simulink model "MAPH_Test"  (R2016a)
settings: Solver=FixedStepDiscrete  StartTime=0.0  StopTime=16  FixedStep=0.005  RelTol=1e-3
undefined symbols (not defined in the file): sigbuilder_block
libraries: MAPH x1
settings Model: Creator=oelkawok  LastModifiedBy=oelkawok
settings DataIOCC: SaveOutput=off  SaveTime=off

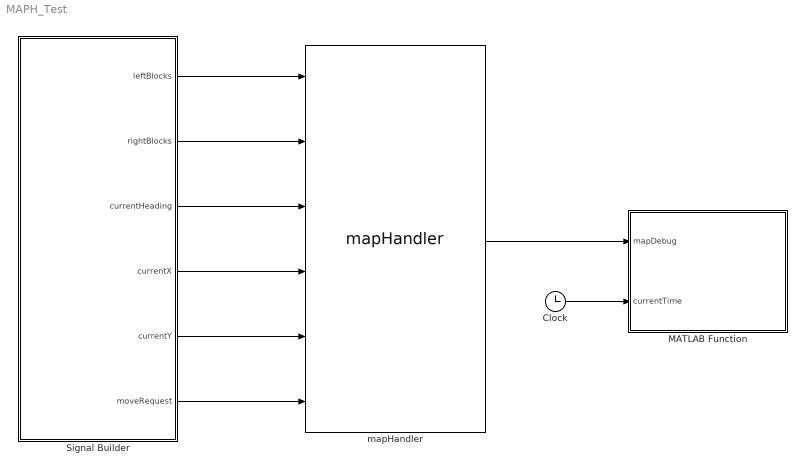
== system MAPH_Test ==
  Clock : Clock
  MATLAB Function : MATLAB Function  TreatAsAtomicUnit=on
  Signal Builder : Subsystem  Tag=STV Subsys  LoadFcn=sigbuilder_block('load',[-655.8 111.6 550.8 400.2 ]);  StartFcn=sigbuilder_block('start');  StopFcn=sigbuilder_block('stop');  ClipboardFcn=sigbuilder_block('clipboard');  mask(Sigbuilder block){}
      mask help: Simulink:masks:SigbuilderBlock_MD
      mask init:
      | if ~strcmp(get_param(bdroot(gcbh),'SimulationStatus'),'stopped') tuvar = sigbuilder_block('maskInit'); end
      settings: CopyFcn=sigbuilder_block('copy');  DeleteFcn=sigbuilder_block('delete');  ModelCloseFcn=sigbuilder_block('modelClose');  PreSaveFcn=sigbuilder_block('preSave');  PauseFcn=sigbuilder_block('pause');  ContinueFcn=sigbuilder_block('continue');  NameChangeFcn=sigbuilder_block('namechange');  OpenFcn=sigbuilder_block('open',[437.6 199.2 550.4 400 ]);  CloseFcn=sigbuilder_block('close');
      mask Display: plot(0, 0, 100, 100,[2, 2, 32, 32, 2], [68, 8, 8, 68, 68],[32, 2], [38, 38], [32, 19, 2],[53, 60, 44], [32, 17, 17, 2],[16, 16, 31, 31]);txt = getActiveGroup(gcbh);text(2, 100, txt,'verticalAlignment', 'top');
  mapHandler : MAPH/mapHandler
  wires:
  mapHandler/1 -> MATLAB Function/1(mapDebug)
  Clock/1 -> MATLAB Function/2(currentTime)
  Signal Builder/3(currentHeading) -> mapHandler/3
  Signal Builder/1(leftBlocks) -> mapHandler/1
  Signal Builder/4(currentX) -> mapHandler/4
  Signal Builder/5(currentY) -> mapHandler/5
  Signal Builder/2(rightBlocks) -> mapHandler/2
  Signal Builder/6(moveRequest) -> mapHandler/6

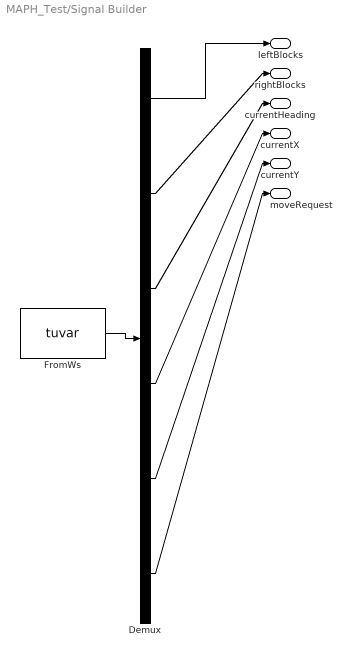
== system MAPH_Test/Signal Builder ==
  Demux : Demux  Tag=STV Demux  Outputs=6
  FromWs : FromWorkspace  Tag=STV FromWs  VariableName=tuvar  SampleTime=0
      SigBuilderData=|
      | common.afterFinalStr = 'Extrapolate'
      | common.sampleTime = 0
      | dataSet(1).timeRange = [0 10]
      | dataSet(1).name = 'Group 1'
      | dataSet(2).timeRange = [0 16]
      | dataSet(2).name = 'UturnRight'
      | dataSet(3).timeRange = [0 16]
      | dataSet(3).name = 'Move_Uturn_right'
      | sbobj.Groups(1).Name = 'Group 1'
      | sbobj.Groups(1).Signals(1).Name = 'leftBlocks'
      | sbobj.Groups(1).Signals(1).XData = [0 4.98 4.98 10]
      | sbobj.Groups(1).Signals(1).YData = [1 1 5 5]
      | sbobj.Groups(1).Signals(2).Name = 'rightBlocks'
      | sbobj.Groups(1).Signals(2).XData = [0 4.98 4.98 10]
      | sbobj.Groups(1).Signals(2).YData = [3 3 4 4]
      | sbobj.Groups(1).Signals(3).Name = 'currentHeading'
      | sbobj.Groups(1).Signals(3).XData = [0 0.4 0.4 5 5 10]
      | sbobj.Groups(1).Signals(3).YData = [400 400 270 270 0 0]
      | sbobj.Groups(1).Signals(4).Name = 'currentX'
      | sbobj.Groups(1).Signals(4).XData = [0 5 5 10]
      | sbobj.Groups(1).Signals(4).YData = [10 10 11 11]
      | sbobj.Groups(1).Signals(5).Name = 'currentY'
      | sbobj.Groups(1).Signals(5).XData = [0 5 10]
      | sbobj.Groups(1).Signals(5).YData = [12 12 12]
      | sbobj.Groups(1).Signals(6).Name = 'moveRequest'
      | sbobj.Groups(1).Signals(6).XData = [0 6.4 6.4 9.6 9.6 16]
      | sbobj.Groups(1).Signals(6).YData = [0 0 1 1 0 0]
      | sbobj.Groups(2).Name = 'UturnRight'
      | sbobj.Groups(2).Signals(1).Name = 'leftBlocks'
      | sbobj.Groups(2).Signals(1).XData = [0 4.98 4.98 7.56 7.56 16]
      | sbobj.Groups(2).Signals(1).YData = [1 1 5 5 6 6]
      | sbobj.Groups(2).Signals(2).Name = 'rightBlocks'
      | sbobj.Groups(2).Signals(2).XData = [0 4.98 4.98 6.48 6.48 7.56 7.56 16]
      | sbobj.Groups(2).Signals(2).YData = [3 3 4 4 2 2 1 1]
      | sbobj.Groups(2).Signals(3).Name = 'currentHeading'
      | sbobj.Groups(2).Signals(3).XData = [0 0.4 0.4 5 6.75 6.75 7 7 7.55 7.55 7.85 7.85 16]
      | sbobj.Groups(2).Signals(3).YData = [400 400 90 90 90 400 400 180 180 400 400 270 270]
      | sbobj.Groups(2).Signals(4).Name = 'currentX'
      | sbobj.Groups(2).Signals(4).XData = [0 5 16]
      | sbobj.Groups(2).Signals(4).YData = [10 10 10]
      | sbobj.Groups(2).Signals(5).Name = 'currentY'
      | sbobj.Groups(2).Signals(5).XData = [0 5 5 7.56 7.56 16]
      | sbobj.Groups(2).Signals(5).YData = [12 12 13 13 12 12]
      | sbobj.Groups(2).Signals(6).Name = 'moveRequest'
      | sbobj.Groups(2).Signals(6).XData = [0 6.74 6.74 7.86 7.86 16]
      | sbobj.Groups(2).Signals(6).YData = [1 1 24 24 1 1]
      | sbobj.Groups(2).TimeRange = [0 16]
      | sbobj.Groups(3).Name = 'Move_Uturn_right'
      | sbobj.Groups(3).Signals(1).Name = 'leftBlocks'
      | sbobj.Groups(3).Signals(1).XData = [0 4.98 4.98 7.56 7.56 16]
      | sbobj.Groups(3).Signals(1).YData = [1 1 5 5 6 6]
      | sbobj.Groups(3).Signals(2).Name = 'rightBlocks'
      | sbobj.Groups(3).Signals(2).XData = [0 4.98 4.98 6.48 6.48 7.56 7.56 16]
      | sbobj.Groups(3).Signals(2).YData = [3 3 4 4 2 2 1 1]
      | sbobj.Groups(3).Signals(3).Name = 'currentHeading'
      | sbobj.Groups(3).Signals(3).XData = [0 0.4 0.4 5 6.75 6.75 7 7 7.55 7.55 7.85 7.85 16]
      | sbobj.Groups(3).Signals(3).YData = [400 400 90 90 90 400 400 180 180 400 400 270 270]
      | sbobj.Groups(3).Signals(4).Name = 'currentX'
      | sbobj.Groups(3).Signals(4).XData = [0 5 7.15 7.15 8.95 16]
      | sbobj.Groups(3).Signals(4).YData = [10 10 10 9 9 9]
      | sbobj.Groups(3).Signals(5).Name = 'currentY'
      | sbobj.Groups(3).Signals(5).XData = [0 5 5 7.56 8.85 8.85 12.1 12.1 16]
      | sbobj.Groups(3).Signals(5).YData = [12 12 13 13 13 12 12 11 11]
      | sbobj.Groups(3).Signals(6).Name = 'moveRequest'
      | sbobj.Groups(3).Signals(6).XData = [0 6.74 6.74 8 8 16]
      | sbobj.Groups(3).Signals(6).YData = [1 1 24 24 1 1]
      | sbobj.Groups(3).TimeRange = [0 16]
  leftBlocks : Outport  Tag=STV Outport
  rightBlocks : Outport  Tag=STV Outport  Port=2
  currentHeading : Outport  Tag=STV Outport  Port=3
  currentX : Outport  Tag=STV Outport  Port=4
  currentY : Outport  Tag=STV Outport  Port=5
  moveRequest : Outport  Tag=STV Outport  Port=6
  wires:
  Demux/1 -> leftBlocks/1
  FromWs/1 -> Demux/1
  Demux/2 -> rightBlocks/1
  Demux/3 -> currentHeading/1
  Demux/4 -> currentX/1
  Demux/5 -> currentY/1
  Demux/6 -> moveRequest/1

== matlab function MAPH_Test/MATLAB Function ==
  data: mapDebug input; currentTime input
function fcn(mapDebug, currentTime)
%#codegen
persistent oldTime;
if isempty(oldTime)
    oldTime = 0;
end

deltaT = currentTime - oldTime;

if(deltaT >= 1)
    oldTime = currentTime;
    hold off;
    clf
    empty = 3;
    uncovered = 1;
    busy = 4;
    hold on
    for i = 1:length(mapDebug(1, :))
        for j = 1:length(mapDebug(1, :))
            if mapDebug(j, i) == empty
                plot(j-1, i-1, '*');
            else if mapDebug(j,i) == busy
                    plot(j-1, i-1, 'o');
                else if mapDebug(j,i) == uncovered
                        plot(j-1, i-1, '.');
                    else
                        plot(j-1, i-1, 'x');
                    end
                end
            end
            
        end
    end
    axis ij
    hold off;
end
